simulink model "cartpend_simulator_2021"  (R2021b)
settings: Solver=ode45  StartTime=0  StopTime=10  MaxStep=0.02  RelTol=1e-3  AbsTol=1e-6
undefined symbols (not defined in the file): F, pend_length, position_init, theta_init
Description:
  | Inverted Pendulum with Animation
  | 
  | This example shows how to model an inverted pendulum.  The animation is created using MATLAB(R) Handle Graphics(R).  The animation block is a masked
  | S-function.  For more information, use the context menu to look under the Animation block's mask
  | and open the S-function for editing.
settings Model: Creator=The MathWorks, Inc.  LastModifiedBy=yamauchi
settings SolverCC: AutoScaleAbsTol=off  AlgebraicLoopSolver=TrustRegion
settings DataIOCC: ExternalInput=[]  InitialState=[]  SaveFormat=Array  SaveOutput=off  SaveTime=off
settings OptimizationCC: BlockReduction=off  BooleanDataType=off  ExpressionDepthLimit=2147483647  InitFltsAndDblsToZero=on  LifeSpan=inf
settings DebuggingCC: SaveWithParameterizedLinksMsg=none  UnderspecifiedInitializationDetection=Classic  MergeDetectMultiDrivingBlocksExec=none  SignalResolutionControl=TryResolveAllWithWarning  MultiTaskDSMMsg=warning  MultiTaskCondExecSysMsg=none  SigSpecEnsureSampleTimeMsg=none  FcnCallInpInsideContextMsg=warning  StateNameClashWarn=warning  SFUnexpectedBacktrackingDiag=warning  SFNoUnconditionalDefaultTransitionDiag=warning  SFExecutionAtInitializationDiag=none  SFMachineParentedDataDiag=warning  ArithmeticOperatorsInVariantConditions=warning
settings HardwareCC: ProdBitPerPointer=32  ProdBitPerSizeT=32  ProdBitPerPtrDiffT=32  ProdLargestAtomicFloat=None  ProdIntDivRoundTo=Undefined  ProdEndianess=Unspecified  ProdWordSize=32  ProdHWDeviceType=32-bit Generic  TargetUnknown=on
settings ModelReferenceCC: PropagateSignalLabelsOutOfModel=off
settings SFSimCC: SimUseLocalCustomCode=off  CustomCodeUndefinedFunction=UseInterfaceOnly
settings RTWCC: RTWUseLocalCustomCode=off
settings CodeAppCC: StateflowObjectComments=on
settings GRTTargetCC: TargetFcnLib=ansi_tfl_tmw.mat  TargetLangStandard=C89/C90 (ANSI)  CombineOutputUpdateFcns=off  GRTInterface=on
settings ConfigComp: CovMetricSettings=dw  CovSaveCumulativeToWorkspaceVar=on  CovSaveSingleToWorkspaceVar=on  CovExternalEMLEnable=off

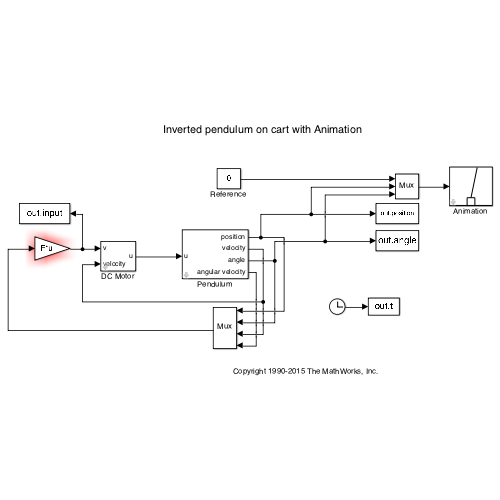
[thumbnail: Simulink's stored preview of the top-level diagram]
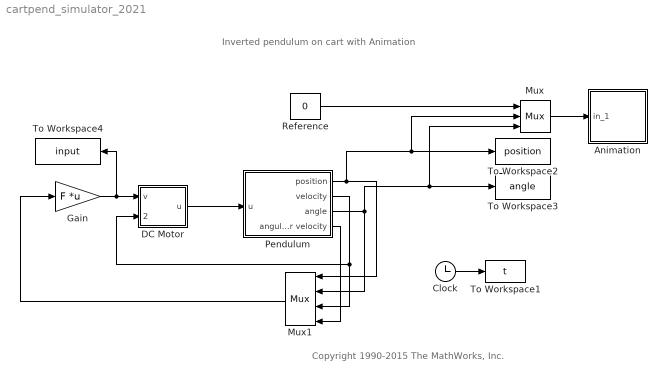
== system cartpend_simulator_2021 ==
  note: Inverted pendulum on cart with Animation
  note: Copyright 1990-2015 The MathWorks, Inc.
  Animation : Subsystem  mask(Pendulum plot){RefBlock=Reference}
      mask prompts: RefBlock "DC reference signal block name:"
      mask help: Pendulum plot
      mask Help: Pendulum animation function using Handle graphics.
      mask Display: plot([-10 10],[0 0],[-2 -2 2 2],[0 1 1 0],[0 3],[1 5])
  Clock : Clock
  DC Motor : Subsystem  mask(Inverted pendulum on cart){Kg=1, Ke=0.023, rho=0.00635, R=8.3}
      mask prompts: Kg "Gear ratio"; Ke "Back-emf constant (V/(rad/s))"; rho "Radius of pinion gear (m)"; R "Armature resistance (Ohm)"
      mask help: Unmask and double-click to see dynamics
      mask Help: Nonlinear dynamics of inverted pendulum on cart.
  Gain : Gain  Gain=F  Multiplication=Matrix(K*u)
  Mux : Mux  Inputs=3
  Mux1 : Mux
  Pendulum : Subsystem  mask(Inverted pendulum on cart){Mcart=0.95, m=0.0568, l=pend_length/2, g=9.8, Dx=1.3, Dt=0.0001}
      mask prompts: Mcart "Mass of cart (kg):"; m "Mass of pendulum (kg):"; l "Distance to pendulum center of mass(m):"; g "Acceleration of gravity (m/s^2):"; Dx "(kg/s)"
      mask help: Unmask and double-click to see dynamics
      mask Help: Nonlinear dynamics of inverted pendulum on cart.
  Reference : Constant  Value=0
  To Workspace1 : ToWorkspace  VariableName=t  SampleTime=-1
      settings: Save2DSignal=2-D array (concatenate along first dimension)
  To Workspace2 : ToWorkspace  VariableName=position  SampleTime=-1
      settings: Save2DSignal=2-D array (concatenate along first dimension)
  To Workspace3 : ToWorkspace  VariableName=angle  SampleTime=-1
      settings: Save2DSignal=2-D array (concatenate along first dimension)
  To Workspace4 : ToWorkspace  VariableName=input  SampleTime=-1
      settings: Save2DSignal=2-D array (concatenate along first dimension)
  wires:
  Mux/1 -> Animation/1(in_1)
  Pendulum/2(velocity) -> Mux1/3, DC Motor/2(velocity)
  Pendulum/4(angular velocity) -> Mux1/4
  Mux1/1 -> Gain/1
  Gain/1 -> To Workspace4/1, DC Motor/1(v)
  Reference/1 -> Mux/1
  Pendulum/1(position) -> To Workspace2/1, Mux/2, Mux1/1
  Pendulum/3(angle) -> Mux1/2, To Workspace3/1, Mux/3
  DC Motor/1(u) -> Pendulum/1(u)
  Clock/1 -> To Workspace1/1

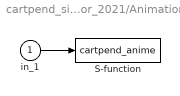
== system cartpend_simulator_2021/Animation ==
  in_1 : Inport
  S-function : S-Function  FunctionName=cartpend_anime  Parameters=RefBlock  SFunctionDeploymentMode=off  EnableBusSupport=off
      settings: DeleteFcn=pendan([],[],[],'DeleteBlock');
  wires:
  in_1/1 -> S-function/1

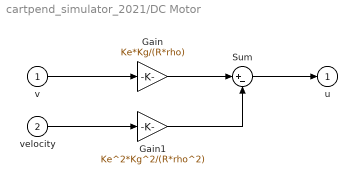
== system cartpend_simulator_2021/DC Motor ==
  v : Inport
  velocity : Inport  Port=2
  Gain : Gain  Gain=Ke*Kg/(R*rho)
  Gain1 : Gain  Gain=Ke^2*Kg^2/(R*rho^2)
  Sum : Sum  Inputs=|+-
  u : Outport  InitialOutput=0  VectorParamsAs1DForOutWhenUnconnected=off
  wires:
  Sum/1 -> u/1
  v/1 -> Gain/1
  velocity/1 -> Gain1/1
  Gain/1 -> Sum/1
  Gain1/1 -> Sum/2

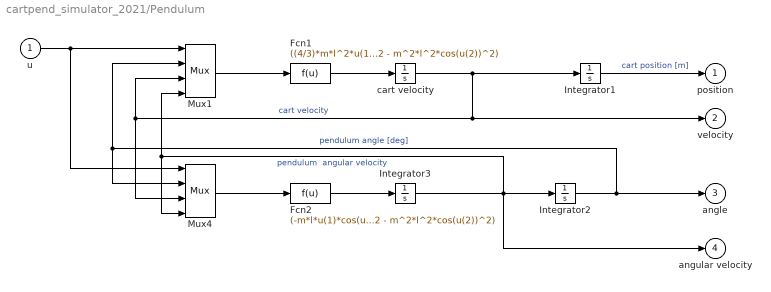
== system cartpend_simulator_2021/Pendulum ==
  u : Inport
  Fcn1 : Fcn  Expr=((4/3)*m*l^2*u(1) + (4/3)*m^2*l^3*u(4)^2*sin(u(2)) - (4/3)*m*l^2*Dx*u(3) - m^2*g*l^2*sin(u(2))*cos(u(2)) + Dt*m*l*u(4)*cos(u(2)))/((4/3)*(Mcart+m)*m*l^2 - m^2*l^2*cos(u(2))^2)
  Fcn2 : Fcn  Expr=(-m*l*u(1)*cos(u(2)) - m^2*l^2*u(4)^2*sin(u(2))*cos(u(2)) + Dx*m*l*u(3)*cos(u(2)) + (Mcart+m)*m*g*l*sin(u(2)) - (Mcart+m)*Dt*u(4))/((4/3)*(Mcart+m)*m*l^2 - m^2*l^2*cos(u(2))^2)
  Integrator1 : Integrator  InitialCondition=position_init
  Integrator2 : Integrator  InitialCondition=theta_init
  Integrator3 : Integrator
  Mux1 : Mux
  Mux4 : Mux
  cart velocity : Integrator
  position : Outport  InitialOutput=0  VectorParamsAs1DForOutWhenUnconnected=off
  velocity : Outport  Port=2  InitialOutput=0  VectorParamsAs1DForOutWhenUnconnected=off
  angle : Outport  Port=3  InitialOutput=0  VectorParamsAs1DForOutWhenUnconnected=off
  angular velocity : Outport  Port=4  InitialOutput=0  VectorParamsAs1DForOutWhenUnconnected=off
  wires:
  Integrator1/1 -> position/1  "cart position [m]"
  Fcn2/1 -> Integrator3/1
  Fcn1/1 -> cart velocity/1
  cart velocity/1 -> velocity/1, Mux1/3, Mux4/3, Integrator1/1  "cart velocity"
  Integrator2/1 -> Mux4/2, Mux1/2, angle/1  "pendulum angle [deg]"
  u/1 -> Mux4/1, Mux1/1
  Mux1/1 -> Fcn1/1
  Mux4/1 -> Fcn2/1
  Integrator3/1 -> angular velocity/1, Mux4/4, Mux1/4, Integrator2/1  "pendulum  angular velocity"
